simulink model "QNX_Node_Train"  (R2026a)
settings: Solver=VariableStepAuto
settings Model: DataDictionary=Architecture_DD.sldd  Creator=jaime  LastModifiedBy=jaime

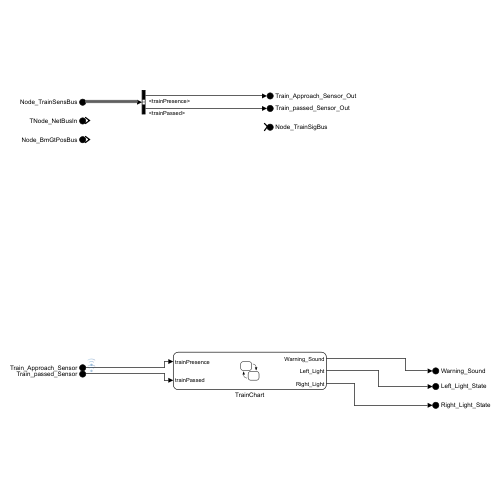
[thumbnail: Simulink's stored preview of the top-level diagram]
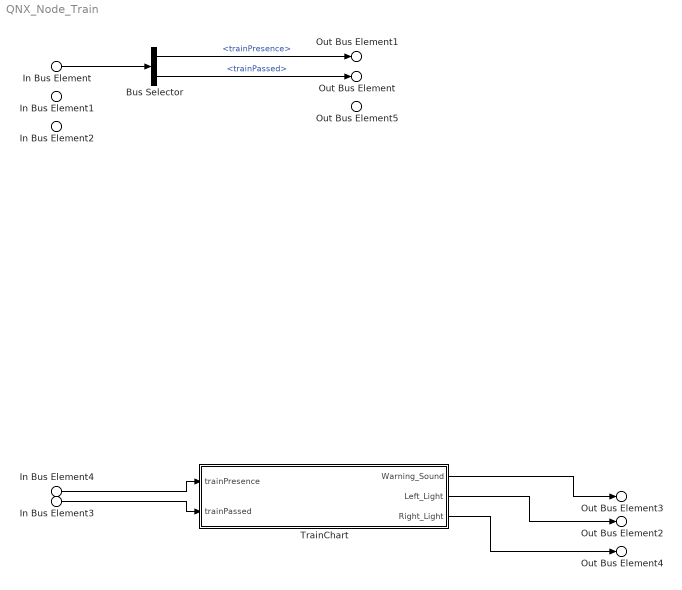
== system QNX_Node_Train ==
  In Bus Element : Inport  PortName=Node_TrainSensBus
  In Bus Element1 : Inport  Port=2  PortName=TNode_NetBusIn
  In Bus Element2 : Inport  Port=3  PortName=Node_BmGtPosBus
  In Bus Element3 : Inport  Port=4  PortName=Train_passed_Sensor
  In Bus Element4 : Inport  Port=5  PortName=Train_Approach_Sensor
  Bus Selector : BusSelector  OutputSignals=trainPresence,trainPassed
  TrainChart : Stateflow chart  TreatAsAtomicUnit=on
  Out Bus Element : Outport  PortName=Train_passed_Sensor_Out
  Out Bus Element1 : Outport  Port=2  PortName=Train_Approach_Sensor_Out
  Out Bus Element3 : Outport  Port=3  PortName=Warning_Sound
  Out Bus Element2 : Outport  Port=4  PortName=Left_Light_State
  Out Bus Element4 : Outport  Port=5  PortName=Right_Light_State
  Out Bus Element5 : Outport  Port=6  PortName=Node_TrainSigBus
  wires:
  In Bus Element/1 -> Bus Selector/1
  Bus Selector/1 -> Out Bus Element1/1  "<trainPresence>"
  Bus Selector/2 -> Out Bus Element/1  "<trainPassed>"
  TrainChart/1(Warning_Sound) -> Out Bus Element3/1
  TrainChart/2(Left_Light) -> Out Bus Element2/1
  TrainChart/3(Right_Light) -> Out Bus Element4/1
  In Bus Element4/1 -> TrainChart/1(trainPresence)
  In Bus Element3/1 -> TrainChart/2(trainPassed)

== stateflow chart QNX_Node_Train/TrainChart ==
  state Idle
    Left_Light = 0
    Right_Light = 0
    Warning_Sound = 0
  state LightState1
    Left_Light = 1
    Right_Light = 0
    Warning_Sound = 1
  state LightState2
    Left_Light = 0
    Right_Light = 1
    Warning_Sound = 1
  (default) -> Idle
  Idle -> LightState1 : [trainPresence == 1]
  LightState1 -> Idle [order 2] : [trainPassed == 1]
  LightState2 -> Idle [order 2] : [trainPassed == 1]
  LightState2 -> LightState1 [order 1] : [after(1, sec)&&(trainPassed ~= 1)]
  LightState1 -> LightState2 [order 1] : [after(1, sec)&&(trainPassed ~= 1)]
  data: Warning_Sound output; trainPresence input; trainPassed input; Left_Light output; Right_Light output
